simulink model "ae2e2"  (R2022a)
settings: Solver=VariableStepAuto  StartTime=0.0  StopTime=inf  RelTol=1e-3
settings Model: Creator=attit  LastModifiedBy=attit

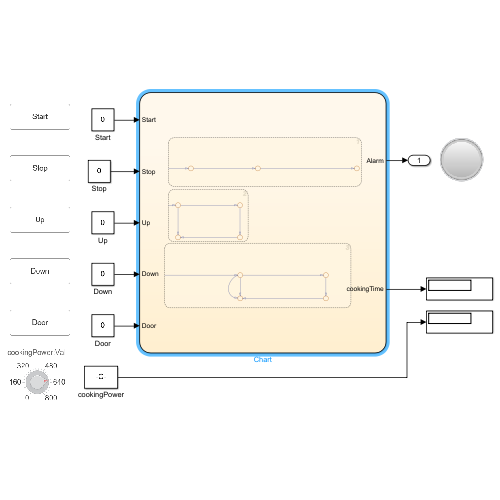
[thumbnail: Simulink's stored preview of the top-level diagram]
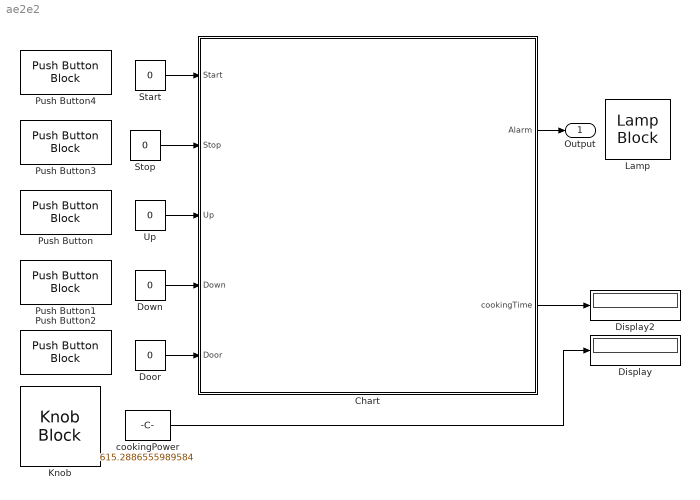
== system ae2e2 ==
  Chart : Stateflow chart  TreatAsAtomicUnit=on
  Display : Display
  Display2 : Display
  Door : Constant  Value=0  OutDataTypeStr=boolean
  Down : Constant  Value=0  OutDataTypeStr=boolean
  Knob : KnobBlock  ScaleMax=800
  Lamp : LampBlock  LabelPosition=Hide
  Push Button : PushButtonBlock  ButtonText=Up  OffValue=0.000000
  Push Button1 : PushButtonBlock  ButtonText=Down  OffValue=0.000000
  Push Button2 : PushButtonBlock  ButtonText=Door  OffValue=0.000000
  Push Button3 : PushButtonBlock  ButtonText=Stop  OffValue=0.000000
  Push Button4 : PushButtonBlock  ButtonText=Start  OffValue=0.000000
  Start : Constant  Value=0  OutDataTypeStr=boolean
  Stop : Constant  Value=0  OutDataTypeStr=boolean
  Up : Constant  Value=0  OutDataTypeStr=boolean
  cookingPower : Constant  Value=615.2886555989584  OutDataTypeStr=uint16
  Output : Outport
  wires:
  cookingPower/1 -> Display/1
  Up/1 -> Chart/3(Up)
  Down/1 -> Chart/4(Down)
  Door/1 -> Chart/5(Door)
  Chart/1(Alarm) -> Output/1
  Stop/1 -> Chart/2(Stop)
  Start/1 -> Chart/1(Start)
  Chart/2(cookingTime) -> Display2/1

== stateflow chart ae2e2/Chart ==
  state oven [parallel]
    du:
    ticks=mod(ticks+1,11)
    settings: executionOrder=1
    oven -> (junction 437)
    (junction 437) -> (junction 441) : [ticks >=10&&cooking==true]
        | {cookingTime=cookingTime-1;
        | ticks = 0;}
    (junction 441) -> (junction 554) : [cooking==true&&cookingTime==0]{Alarm=true}
  state Oven [parallel]
    en,du:
    settings: executionOrder=2
    Oven -> (junction 251)
    (junction 251) -> (junction 257) [order 1] : [Up==1]
        | {cookingTime=cookingTime+30}
    (junction 251) -> (junction 255) [order 2] : [Down==1]
        | {cookingTime=cookingTime-30}
    (junction 257) -> (junction 263)
    (junction 263) -> (junction 255)
  state Cooking [parallel]
    du:
    settings: executionOrder=3
    Cooking -> (junction 279)
    (junction 279) -> (junction 297) [order 1] : [Door==0&&Start==1]{cooking=true;
        | cookingTime;}
    (junction 279) -> (junction 283) [order 3] : [Door==1]{cooking=false;
        | cookingTime=cookingTime-1}
    (junction 279) -> (junction 283) [order 2] : [Door==0&&Stop==1]
        | {cooking=false;
        | cookingTime==cookingTime-1;Alarm=false;}
    (junction 297) -> (junction 299)
    (junction 299) -> (junction 283)
  data: Start input boolean; Stop input boolean; Up input boolean; Down input boolean; Alarm output boolean =false; Door input boolean; cooking local boolean =false; cookingTime output uint16 [0..] =uint16(0); ticks local uint16 =uint16(0)
